simulink model "SensorInputs"  (R2024b)
settings: Solver=FixedStepAuto  StartTime=0.0  StopTime=10.0  RelTol=1e-3  EnableMultiTasking=on
settings Model: DataDictionary=Master_Dictionary.sldd  EnableAccessToBaseWorkspace=off  Creator=torni  LastModifiedBy=Will
settings OptimizationCC: DefaultParameterBehavior=Inlined  EnhancedBackFolding=on  PassReuseOutputArgsAs=Individual arguments  ZeroExternalMemoryAtStartup=off  ZeroInternalMemoryAtStartup=off  MaxStackSize=8192  OptimizeBlockOrder=speed  DifferentSizesBufferReuse=on  OptimizationCustomize=off  EfficientTunableParamExpr=on
settings DebuggingCC: ParameterTunabilityLossMsg=error
settings HardwareCC: ProdBitPerPointer=32  ProdBitPerSizeT=32  ProdBitPerPtrDiffT=32  ProdLargestAtomicInteger=Long  ProdLargestAtomicFloat=Double  ProdWordSize=32  ProdLongLongMode=on  ProdHWDeviceType=ARM Compatible->ARM Cortex-M
settings SFSimCC: MATLABDynamicMemAlloc=off
settings RTWCC: Description=Embedded Coder  SystemTargetFile=ert.tlc  HardwareBoard=STM32H7xx Based (Single-core)  TemplateMakefile=ert_default_tmf  Toolchain=GNU Tools for ARM Embedded Processors
settings CodeAppCC: ForceParamTrailComments=on  IgnoreCustomStorageClasses=off  OperatorAnnotations=on  SimulinkDataObjDesc=on  SFDataObjDesc=on  InsertBlockDesc=on
settings ERTTargetCC: TargetLangStandard=C99 (ISO)  CodeReplacementLibrary=ARM Cortex-M  ExtModeTransport=3  ExtModeStaticAlloc=on  ExtModeStaticAllocSize=2048  ExtModeMexFile=ext_xcp  ExtModeIntrfLevel=Level2 - Open

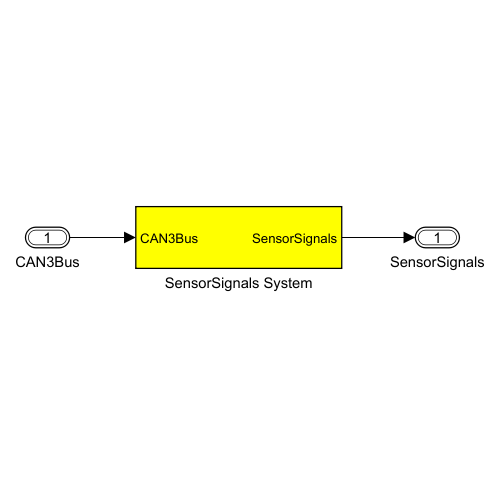
[thumbnail: Simulink's stored preview of the top-level diagram]
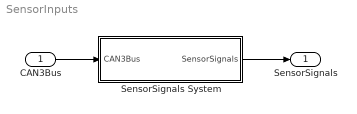
== system SensorInputs ==
  CAN3Bus : Inport  OutDataTypeStr=Bus: CAN3Bus
  SensorSignals System : Subsystem
  SensorSignals : Outport  OutDataTypeStr=Bus: SensorSignals  VectorParamsAs1DForOutWhenUnconnected=off
  wires:
  CAN3Bus/1 -> SensorSignals System/1(CAN3Bus)
  SensorSignals System/1(SensorSignals) -> SensorSignals/1

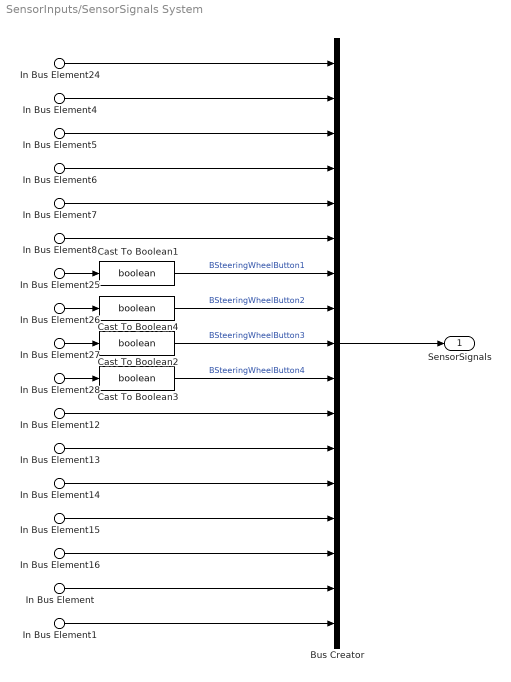
== system SensorInputs/SensorSignals System ==
  In Bus Element5 : Inport  PortName=CAN3Bus  Element=DDU7.NDisplayNumberDDU7
  In Bus Element6 : Inport  PortName=CAN3Bus  Element=DDU7.VSteeringAngle
  In Bus Element7 : Inport  PortName=CAN3Bus  Element=DDU7.VThrottlePedal1
  In Bus Element8 : Inport  PortName=CAN3Bus  Element=DDU7.VThrottlePedal2
  In Bus Element : Inport  PortName=CAN3Bus  Element=DDU7.VBrakeF
  In Bus Element1 : Inport  PortName=CAN3Bus  Element=DDU7.VBrakeR
  In Bus Element4 : Inport  PortName=CAN3Bus  Element=DDU7.VDamperPotentiometerFR
  In Bus Element24 : Inport  PortName=CAN3Bus  Element=DDU7.VDamperPotentiometerFL
  In Bus Element25 : Inport  PortName=CAN3Bus  Element=STW.BSteeringWheelButton1
  In Bus Element26 : Inport  PortName=CAN3Bus  Element=STW.BSteeringWheelButton2
  In Bus Element27 : Inport  PortName=CAN3Bus  Element=STW.BSteeringWheelButton3
  In Bus Element28 : Inport  PortName=CAN3Bus  Element=STW.BSteeringWheelButton4
  In Bus Element12 : Inport  PortName=CAN3Bus  Element=STW.NPageSelectRotary
  In Bus Element13 : Inport  PortName=CAN3Bus  Element=STW.NParameterRotary
  In Bus Element14 : Inport  PortName=CAN3Bus  Element=STW.NEventModeRotary
  In Bus Element15 : Inport  PortName=CAN3Bus  Element=STW.VRegenPaddle1
  In Bus Element16 : Inport  PortName=CAN3Bus  Element=STW.VRegenPaddle2
  Bus Creator : BusCreator  Inputs=17  OutDataTypeStr=Bus: SensorSignals  NonVirtualBus=on
  Cast To Boolean{1..4} (4 alike) : DataTypeConversion  OutDataTypeStr=boolean  SaturateOnIntegerOverflow=off  RndMeth=Floor
  SensorSignals : Outport  OutDataTypeStr=Bus: SensorSignals  VectorParamsAs1DForOutWhenUnconnected=off  LockScale=on
  wires:
  In Bus Element24/1 -> Bus Creator/1
  In Bus Element5/1 -> Bus Creator/3
  In Bus Element6/1 -> Bus Creator/4
  In Bus Element7/1 -> Bus Creator/5
  In Bus Element8/1 -> Bus Creator/6
  In Bus Element27/1 -> Cast To Boolean2/1
  In Bus Element28/1 -> Cast To Boolean3/1
  In Bus Element12/1 -> Bus Creator/11
  In Bus Element13/1 -> Bus Creator/12
  In Bus Element14/1 -> Bus Creator/13
  In Bus Element15/1 -> Bus Creator/14
  In Bus Element16/1 -> Bus Creator/15
  In Bus Element/1 -> Bus Creator/16
  In Bus Element1/1 -> Bus Creator/17
  Bus Creator/1 -> SensorSignals/1
  In Bus Element4/1 -> Bus Creator/2
  Cast To Boolean1/1 -> Bus Creator/7  "BSteeringWheelButton1"
  Cast To Boolean4/1 -> Bus Creator/8  "BSteeringWheelButton2"
  Cast To Boolean2/1 -> Bus Creator/9  "BSteeringWheelButton3"
  Cast To Boolean3/1 -> Bus Creator/10  "BSteeringWheelButton4"
  In Bus Element25/1 -> Cast To Boolean1/1
  In Bus Element26/1 -> Cast To Boolean4/1
